simulink subsystem "fan"  (R2020b)
settings: Solver=VariableStepAuto  StartTime=0.0  StopTime=10.0  RelTol=1e-3
values from neighbouring files (symbols this model uses):
  CFM2CMS = 0.00047194745    [fan_defs.m]
  rho = 1.225    [heat_sink_defs.m]
  RPM2CFM = readmatrix('CFMvsRPM.csv')    [fan_defs.m]
  tauFan = 0.2192    [fan_defs.m]
  V2RPM = readmatrix('RPMvsV.csv')    [fan_defs.m]
settings Model: Creator=jclinton  LastModifiedBy=jclinton
settings DebuggingCC: SFMachineParentedDataDiag=error

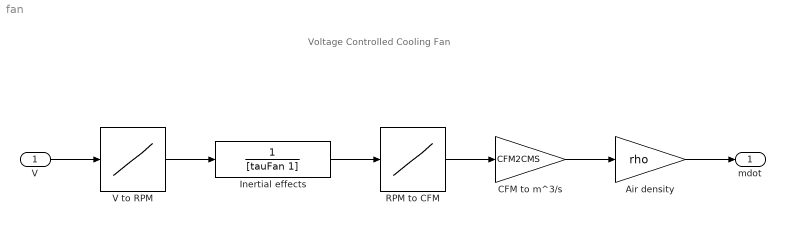
== system fan ==
  note: Voltage Controlled Cooling Fan
  V : Inport  Unit=V
  Air density : Gain  Gain=rho
  CFM to m^3/s : Gain  Gain=CFM2CMS
  Inertial effects : TransferFcn  Denominator=[tauFan 1]
  RPM to CFM : Lookup_n-D  NumberOfTableDimensions=1  BreakpointsForDimension1=RPM2CFM(:,1)  Table=RPM2CFM(:,2)  InternalRulePriority=Speed  RndMeth=Simplest  InputSameDT=on
  V to RPM : Lookup_n-D  NumberOfTableDimensions=1  BreakpointsForDimension1=V2RPM(:,1)  Table=V2RPM(:,2)  InternalRulePriority=Speed  RndMeth=Simplest  InputSameDT=on
  mdot : Outport  Unit=kg/sec
  wires:
  V/1 -> V to RPM/1
  V to RPM/1 -> Inertial effects/1
  Inertial effects/1 -> RPM to CFM/1
  RPM to CFM/1 -> CFM to m^3/s/1
  CFM to m^3/s/1 -> Air density/1
  Air density/1 -> mdot/1
